simulink model "myammod"  (R2014b)
settings: Solver=ode3  StartTime=0.0  StopTime=10.0  FixedStep=.001  RelTol=1e-3
settings Model: Creator=Ben  LastModifiedBy=Ben

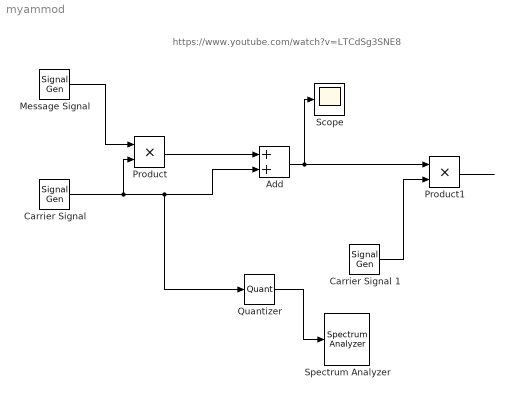
== system myammod ==
  note: https://www.youtube.com/watch?v=LTCdSg3SNE8
  Add : Sum
  "Carrier Signal " : SignalGenerator  Frequency=1500  Units=rad/sec
  Carrier Signal 1 : SignalGenerator  Frequency=1500  Units=rad/sec
  "Message Signal " : SignalGenerator  Amplitude=.7  Frequency=200  Units=rad/sec
  Product : Product
  Product1 : Product
  Quantizer : Quantizer  SampleTime=.001
  Scope : Scope
  Spectrum Analyzer : SpectrumAnalyzer
  wires:
  "Message Signal "/1 -> Product/1
  Product/1 -> Add/1
  "Carrier Signal "/1 -> Product/2, Quantizer/1, Add/2
  Carrier Signal 1/1 -> Product1/2
  Product1/1 -> ?
  Add/1 -> Product1/1, Scope/1
  Quantizer/1 -> Spectrum Analyzer/1
